simulink model "Flipper"  (R2017b)
settings: Solver=VariableStepAuto  StartTime=0.0  StopTime=100.0  RelTol=1e-3
libraries: vrlib x2
settings Model: Creator=aby032  LastModifiedBy=aby032

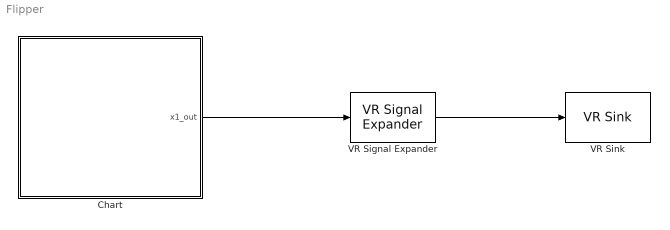
== system Flipper ==
  Chart : Stateflow chart  TreatAsAtomicUnit=on
  VR Signal Expander : vrlib/VR Signal Expander  outwidth=3  outidx=[1 2]
      settings: SourceProductName=Simulink 3D Animation  SourceProductBaseCode=VR
  VR Sink : vrlib/VR Sink  InstantiateOnLoad=on  SampleTime=0.05  ViewEnable=on  RemoteChange=off  RemoteView=off  FieldsWritten=Ball.translation.3.1.1.double  WorldFileName=Table.wrl  AutoView=off  VideoDimensions=[]  AllowVariableSize=off
      settings: SourceProductBaseCode=VR
  wires:
  Chart/1(x1_out) -> VR Signal Expander/1
  VR Signal Expander/1 -> VR Sink/1

== stateflow chart Flipper/Chart ==
  settings: updateMethod=CONTINUOUS
  state Flipper
    during:
    %DGL
    [v1_dot(1),v1_dot(2)] = Acc();
    x1_dot = v1;
    %Output
    x1_out=x1;
  (default) -> Flipper : {Init()}
  Flipper -> Flipper [order 4] : [Wand3Kontakt()]{Wand3Refl();}
  Flipper -> Flipper [order 1] : [Wand1Kontakt()]{Wand1Refl();}
  Flipper -> Flipper [order 2] : [Wand2Kontakt()]{Wand2Refl();}
  Flipper -> Flipper [order 3] : [HndKontakt()]{HndRefl();}
  data: k function_output boolean; ax function_output; ay function_output; k function_output boolean; k function_output boolean; k function_output boolean; R constant double =0.25; RHnd constant double =0.8; Hnd local double size=2,1; n1 local double size=2,1; n2 local double size=2,1; n3 local double size=2,1; p1 local double size=2,1; p2 local double size=2,1; p3 local double size=2,1; p4 local double size=2,1; t1 local double size=2,1; t2 local double size=2,1; t3 local double size=2,1; v1 local double size=2,1; x1 local double size=2,1; x1_out output double size=2,1
  data v1 settings: updateMethod=SF_CONTINUOUS_TIME_DATA
  data x1 settings: updateMethod=SF_CONTINUOUS_TIME_DATA
  function Init:
    | function Init
    |     p1 =  [0; 5];
    |     p2 =  [5; 0];
    |     p3 =  [9; 0];
    |     p4 =  [10; 7];
    | 
    |     Hnd = [6; 2.5];
    | 
    |     x1 = [4; 5];        %Startposition
    |     v1 = [0; 0];        %Startgeschwindigkeit
    | 
    | 
    | 
    |     t1 = (p2-p1)/norm(p2-p1);
    |     n1 = [-t1(2); t1(1)];
    | 
    |     t2 = (p3-p2)/norm(p3-p2);
    |     n2 = [-t2(2); t2(1)];
    | 
    |     t3 = (p4-p3)/norm(p4-p3);
    |     n3 = [-t3(2); t3(1)];
    | end
  function k = Wand1Kontakt:
    | function k = Wand1Kontakt
    |     k = (((x1-p1)' * n1) <= R);
    | end
  function Wand1Refl:
    | function Wand1Refl
    |    v1t = (v1' * t1) * t1;
    |    v1n = -(v1' * n1) * n1;
    |    v1 = v1t + v1n;
    | end
  function [ax, ay] = Acc:
    | function [ax, ay] = Acc
    |     ax = 0;
    |     ay = -1;        %Beschleunigung
    | end
  function k = Wand2Kontakt:
    | function k = Wand2Kontakt
    |     k = ((x1-p2)' * n2) <= R;
    | end
  function Wand2Refl:
    | function Wand2Refl
    |    v1t = (v1' * t2) * t2;
    |    v1n = -(v1' * n2) * n2;
    |    v1 = v1t + v1n;
    | end
  function k = Wand3Kontakt:
    | function k = Wand3Kontakt
    |     k = ((x1-p3)' * n3) <= R;
    | end
  function Wand3Refl:
    | function Wand3Refl
    |    v1t = (v1' * t3) * t3;
    |    v1n = -(v1' * n3) * n3;
    |    v1 = v1t + v1n;
    | end
  function k = HndKontakt:
    | function k = HndKontakt
    |     k = norm(Hnd - x1) <= (R+RHnd);
    | end
  function HndRefl:
    | function HndRefl
    |  n = (x1- Hnd)/norm(x1-Hnd);
    |  t = [n(2);-n(1)];
    |  
    |  v1t = (v1' * t) * t;
    |  v1n = -(v1' * n) * n;
    |  
    |  v1 = v1t + v1n;
    | end
